simulink subsystem "clarktrn"  (R2020a)
settings: Solver=VariableStepAuto  StartTime=0.0  StopTime=10.0  RelTol=1e-3
settings Model: Creator=ZhuanZ（无密码）  LastModifiedBy=ZhuanZ（无密码）

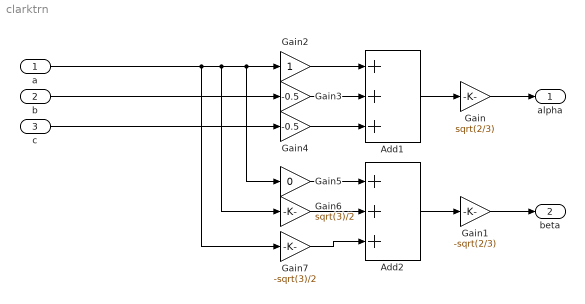
== system clarktrn ==
  a : Inport
  b : Inport  Port=2
  c : Inport  Port=3
  Add1 : Sum  Inputs=+++
  Add2 : Sum  Inputs=+++
  Gain : Gain  Gain=sqrt(2/3)
  Gain1 : Gain  Gain=-sqrt(2/3)
  Gain2 : Gain
  Gain3 : Gain  Gain=-0.5
  Gain4 : Gain  Gain=-0.5
  Gain5 : Gain  Gain=0
  Gain6 : Gain  Gain=sqrt(3)/2
  Gain7 : Gain  Gain=-sqrt(3)/2
  alpha : Outport
  beta : Outport  Port=2
  wires:
  Add1/1 -> Gain/1
  Add2/1 -> Gain1/1
  Gain/1 -> alpha/1
  Gain1/1 -> beta/1
  Gain2/1 -> Add1/1
  a/1 -> Gain7/1, Gain6/1, Gain5/1, Gain2/1
  Gain4/1 -> Add1/3
  Gain3/1 -> Add1/2
  Gain5/1 -> Add2/1
  Gain6/1 -> Add2/2
  Gain7/1 -> Add2/3
  b/1 -> Gain3/1
  c/1 -> Gain4/1
